simulink model "CS2_Hzw"  (R2018b)
settings: Solver=VariableStepAuto  StartTime=0.0  StopTime=10.0  RelTol=1e-3
settings Model: Creator=bogda  LastModifiedBy=bogda

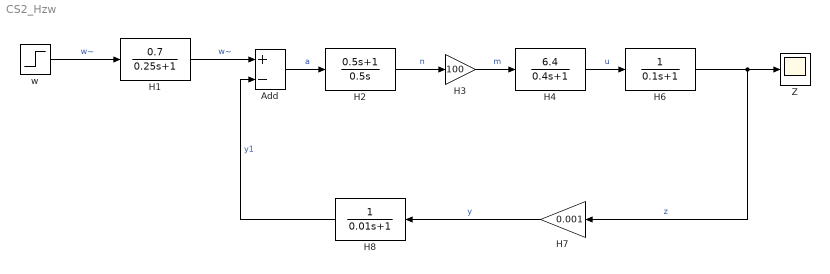
== system CS2_Hzw ==
  Add : Sum  Inputs=+-
  H1 : TransferFcn  Numerator=[0.7]  Denominator=[0.25 1]
  H2 : TransferFcn  Numerator=[0.5 1]  Denominator=[0.5 0]
  H3 : Gain  Gain=100
  H4 : TransferFcn  Numerator=[6.4]  Denominator=[0.4 1]
  H6 : TransferFcn  Denominator=[0.1 1]
  H7 : Gain  Gain=0.001
  H8 : TransferFcn  Denominator=[0.01 1]
  Z : Scope
  w : Step  Time=0  After=10  SampleTime=0
  wires:
  H3/1 -> H4/1  "m"
  H7/1 -> H8/1  "y"
  H4/1 -> H6/1  "u"
  w/1 -> H1/1  "w~"
  Add/1 -> H2/1  "a"
  H1/1 -> Add/1  "w~"
  H8/1 -> Add/2  "y1"
  H2/1 -> H3/1  "n"
  H6/1 -> Z/1, H7/1  "z"
